simulink model "Eg3_6"  (R2018a)
settings: Solver=VariableStepAuto  StartTime=0.0  StopTime=50  RelTol=1e-3
settings Model: Creator=wangluo  LastModifiedBy=wangluo

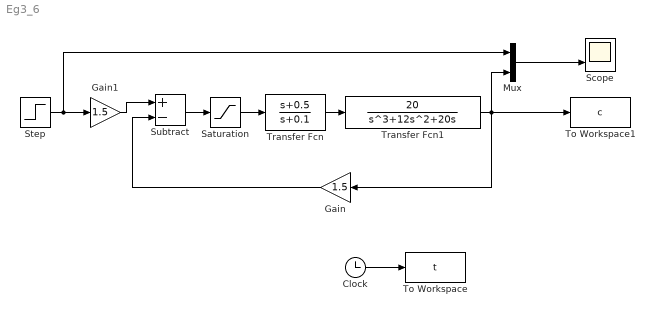
== system Eg3_6 ==
  Clock : Clock
  Gain : Gain  Gain=1.5
  Gain1 : Gain  Gain=1.5
  Mux : Mux  Inputs=2
  Saturation : Saturate  LowerLimit=-0.2
  Scope : Scope  NumInputPorts=2
  Step : Step  SampleTime=0
  Subtract : Sum  Inputs=+-
  To Workspace : ToWorkspace  VariableName=t  SampleTime=-1
  To Workspace1 : ToWorkspace  VariableName=c  SampleTime=-1
  Transfer Fcn : TransferFcn  Numerator=[1 0.5]  Denominator=[1 0.1]
  Transfer Fcn1 : TransferFcn  Numerator=[20]  Denominator=[1 12 20 0]
  wires:
  Transfer Fcn/1 -> Transfer Fcn1/1
  Step/1 -> Gain1/1, Mux/1
  Transfer Fcn1/1 -> To Workspace1/1, Gain/1, Mux/2
  Gain/1 -> Subtract/2
  Clock/1 -> To Workspace/1
  Mux/1 -> Scope/2
  Gain1/1 -> Subtract/1
  Subtract/1 -> Saturation/1
  Saturation/1 -> Transfer Fcn/1
